simulink model "designed_pid"  (R2019b)
settings: Solver=VariableStepAuto  StartTime=0.0  StopTime=10  MaxStep=0.01  RelTol=1e-4  EnableMultiTasking=on
settings Model: Creator=danma  LastModifiedBy=danma
settings DataIOCC: LimitDataPoints=on  SaveOutput=off  SaveTime=off
settings OptimizationCC: ExpressionDepthLimit=2147483647  LifeSpan=1
settings DebuggingCC: UnderspecifiedInitializationDetection=Classic  MergeDetectMultiDrivingBlocksExec=none  FcnCallInpInsideContextMsg=warning  AllowSymbolicDim=off  StateNameClashWarn=warning  SFUnexpectedBacktrackingDiag=warning  SFNoUnconditionalDefaultTransitionDiag=warning  SFExecutionAtInitializationDiag=none  ArithmeticOperatorsInVariantConditions=warning
settings SFSimCC: SimUseLocalCustomCode=off  CustomCodeUndefinedFunction=UseInterfaceOnly
settings RTWCC: RTWUseLocalCustomCode=off
settings CodeAppCC: StateflowObjectComments=on
settings GRTTargetCC: TargetLangStandard=C89/C90 (ANSI)  GeneratePreprocessorConditionals=Disable all  CombineOutputUpdateFcns=off  GRTInterface=on

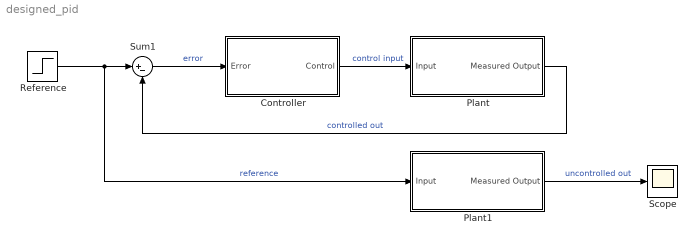
== system designed_pid ==
  Controller : Subsystem
  Plant : Subsystem
  Plant1 : Subsystem
  Reference : Step  Time=0.5  SampleTime=0
  Scope : Scope
  Sum1 : Sum  Inputs=|+-
  wires:
  Controller/1(Control) -> Plant/1(Input)  "control input"
  Sum1/1 -> Controller/1(Error)  "error"
  Plant/1(Measured Output) -> Sum1/2  "controlled out"
  Plant1/1(Measured Output) -> Scope/1  "uncontrolled out"
  Reference/1 -> Plant1/1(Input), Sum1/1  "reference"

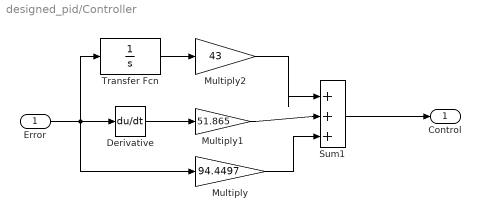
== system designed_pid/Controller ==
  Error : Inport
  Derivative : Derivative
  Multiply : Gain  Gain=94.4497
  Multiply1 : Gain  Gain=51.865
  Multiply2 : Gain  Gain=43
  Sum1 : Sum  Inputs=|+++
  Transfer Fcn : TransferFcn  Denominator=[1 0]
  Control : Outport
  wires:
  Sum1/1 -> Control/1
  Error/1 -> Transfer Fcn/1, Multiply/1, Derivative/1
  Multiply2/1 -> Sum1/1
  Multiply/1 -> Sum1/3
  Multiply1/1 -> Sum1/2
  Transfer Fcn/1 -> Multiply2/1
  Derivative/1 -> Multiply1/1

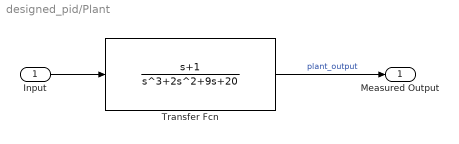
== system designed_pid/Plant ==
  Input : Inport
  Transfer Fcn : TransferFcn  Numerator=[1 1]  Denominator=[1 2 9 20]
  Measured Output : Outport
  wires:
  Input/1 -> Transfer Fcn/1
  Transfer Fcn/1 -> Measured Output/1  "plant_output"

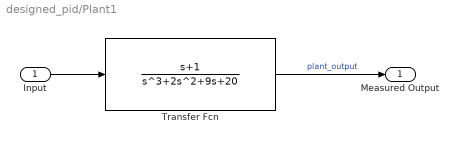
== system designed_pid/Plant1 ==
  Input : Inport
  Transfer Fcn : TransferFcn  Numerator=[1 1]  Denominator=[1 2 9 20]
  Measured Output : Outport
  wires:
  Input/1 -> Transfer Fcn/1
  Transfer Fcn/1 -> Measured Output/1  "plant_output"
